simulink model "cart_pole"  (R2024b)
settings: Solver=ode4  StartTime=0.0  StopTime=t_end  FixedStep=0.001  RelTol=1e-3
values from neighbouring files (symbols this model uses):
  alpha = deg2rad(15)    [init_params.m]
  b = 0.1    [init_params.m]    (also in pendulum.m)
  beta = 1.5    [init_params.m]
  C = 0.001    [init_params.m]    (also in pendulum.m = 0.01)
  g = 9.81    [init_params.m]
  J = (1/3)*m*l^2    (= 0.006)    [init_params.m]    (also in pendulum.m)
  K = lqr(A, B, Q, R)    [init_params.m]
  l = 0.3    [init_params.m]    (also in pendulum.m)
  m = 0.2    [init_params.m]    (also in pendulum.m)
  M_t = M_c + m    (= 1.7)    [init_params.m]
  theta0 = pi - 0.05    (= 3.09159265359)    [init_params.m]    (also in pendulum.m = deg2rad(5))
  theta_dot0 = 0    [init_params.m]
  x0 = 0    [init_params.m]    (also in pendulum.m)
  x_dot0 = 0    [init_params.m]
settings Model: Creator=Ali Emir Kaplan  LastModifiedBy=Ali Emir Kaplan

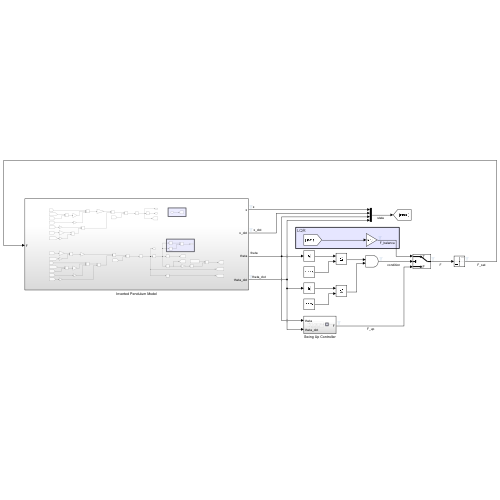
[thumbnail: Simulink's stored preview of the top-level diagram]
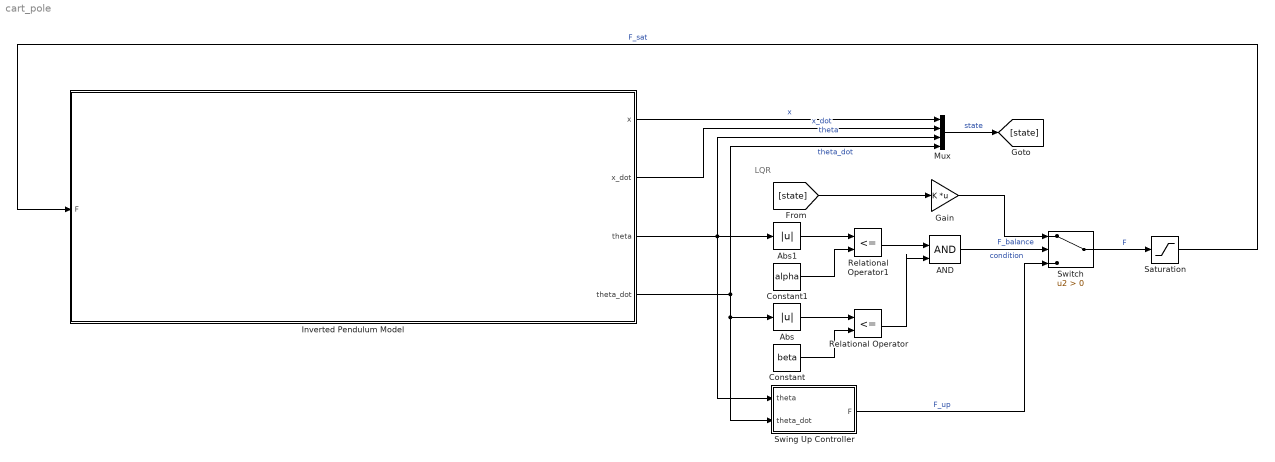
== system cart_pole ==
  note: LQR
  AND : Logic  IconShape=distinctive  AllPortsSameDT=off  OutDataTypeStr=boolean
  Abs : Abs  SaturateOnIntegerOverflow=off
  Abs1 : Abs  SaturateOnIntegerOverflow=off
  Constant : Constant  Value=beta
  Constant1 : Constant  Value=alpha
  Gain : Gain  Gain=K  Multiplication=Matrix(K*u)
  Inverted Pendulum Model : Subsystem
  Mux : Mux
  Relational Operator : RelationalOperator  Operator=<=  OutDataTypeStr=boolean  RndMeth=Simplest  InputSameDT=off
  Relational Operator1 : RelationalOperator  Operator=<=  OutDataTypeStr=boolean  RndMeth=Simplest  InputSameDT=off
  Saturation : Saturate  UpperLimit=+30  LowerLimit=-30
  Swing Up Controller : Subsystem
  Switch : Switch  Criteria=u2 > Threshold  SaturateOnIntegerOverflow=off  InputSameDT=off
  wires:
  Inverted Pendulum Model/1(x) -> Mux/1  "x"
  Inverted Pendulum Model/2(x_dot) -> Mux/2  "x_dot"
  Inverted Pendulum Model/3(theta) -> Mux/3, Abs1/1, Swing Up Controller/1(theta)  "theta"
  Inverted Pendulum Model/4(theta_dot) -> Swing Up Controller/2(theta_dot), Abs/1, Mux/4  "theta_dot"
  Swing Up Controller/1(F) -> Switch/3  "F_up"
  Mux/1 -> [state]  "state"
  [state] -> Gain/1
  Constant/1 -> Relational Operator/2
  Abs/1 -> Relational Operator/1
  Constant1/1 -> Relational Operator1/2
  Abs1/1 -> Relational Operator1/1
  Relational Operator1/1 -> AND/1
  Relational Operator/1 -> AND/2
  Gain/1 -> Switch/1  "F_balance"
  AND/1 -> Switch/2  "condition"
  Switch/1 -> Saturation/1  "F"
  Saturation/1 -> Inverted Pendulum Model/1(F)  "F_sat"

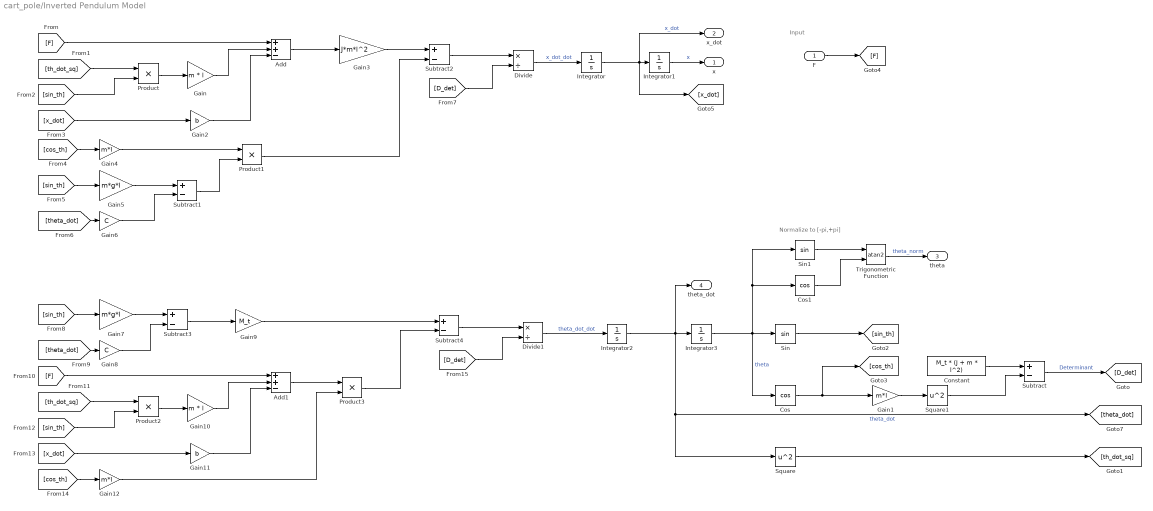
== system cart_pole/Inverted Pendulum Model ==
  note: Input
  note: Normalize to [-pi,+pi]
  F : Inport
  Add : Sum  Inputs=++-
  Add1 : Sum  Inputs=++-
  Constant : Constant  Value=M_t * (J + m * l^2)
  Cos : Trigonometry  Operator=cos
  Cos1 : Trigonometry  Operator=cos
  Divide : Product  Inputs=*/
  Divide1 : Product  Inputs=*/
  Gain : Gain  Gain=m * l
  Gain1 : Gain  Gain=m*l
  Gain10 : Gain  Gain=m * l
  Gain11 : Gain  Gain=b
  Gain12 : Gain  Gain=m*l
  Gain2 : Gain  Gain=b
  Gain3 : Gain  Gain=J*m*l^2
  Gain4 : Gain  Gain=m*l
  Gain5 : Gain  Gain=m*g*l
  Gain6 : Gain  Gain=C
  Gain7 : Gain  Gain=m*g*l
  Gain8 : Gain  Gain=C
  Gain9 : Gain  Gain=M_t
  Integrator : Integrator  InitialCondition=x_dot0
  Integrator1 : Integrator  InitialCondition=x0
  Integrator2 : Integrator  InitialCondition=theta_dot0
  Integrator3 : Integrator  InitialCondition=theta0
  Product{,1..3} (4 alike) : Product
  Sin : Trigonometry
  Sin1 : Trigonometry
  Square : Math  Operator=square
  Square1 : Math  Operator=square
  Subtract{,1..4} (5 alike) : Sum  Inputs=+-
  Trigonometric Function : Trigonometry  Operator=atan2
  x : Outport
  x_dot : Outport  Port=2
  theta : Outport  Port=3
  theta_dot : Outport  Port=4
  wires:
  Integrator1/1 -> x/1  "x"
  Integrator/1 -> x_dot/1, [x_dot], Integrator1/1  "x_dot"
  Divide/1 -> Integrator/1  "x_dot_dot"
  F/1 -> [F]
  [th_dot_sq] -> Product/1
  [sin_th] -> Product/2
  Product/1 -> Gain/1
  Gain/1 -> Add/2
  [F] -> Add/1
  [x_dot] -> Gain2/1
  Gain2/1 -> Add/3
  Add/1 -> Gain3/1
  [cos_th] -> Gain4/1
  [sin_th] -> Gain5/1
  [theta_dot] -> Gain6/1
  Gain5/1 -> Subtract1/1
  Gain6/1 -> Subtract1/2
  Gain4/1 -> Product1/1
  Subtract1/1 -> Product1/2
  Product1/1 -> Subtract2/2
  Gain3/1 -> Subtract2/1
  Subtract2/1 -> Divide/1
  [D_det] -> Divide/2
  [sin_th] -> Gain7/1
  [theta_dot] -> Gain8/1
  Gain7/1 -> Subtract3/1
  Gain8/1 -> Subtract3/2
  Subtract3/1 -> Gain9/1
  Gain11/1 -> Add1/3
  [sin_th] -> Product2/2
  Gain10/1 -> Add1/2
  [F] -> Add1/1
  [th_dot_sq] -> Product2/1
  Product2/1 -> Gain10/1
  [x_dot] -> Gain11/1
  [cos_th] -> Gain12/1
  Add1/1 -> Product3/1
  Gain12/1 -> Product3/2
  Gain9/1 -> Subtract4/1
  Product3/1 -> Subtract4/2
  [D_det] -> Divide1/2
  Subtract4/1 -> Divide1/1
  Divide1/1 -> Integrator2/1  "theta_dot_dot"
  Gain1/1 -> Square1/1
  Integrator2/1 -> theta_dot/1, Square/1, [theta_dot], Integrator3/1  "theta_dot"
  Square/1 -> [th_dot_sq]
  Cos/1 -> [cos_th], Gain1/1
  Integrator3/1 -> Sin1/1, Cos1/1, Cos/1, Sin/1  "theta"
  Constant/1 -> Subtract/1
  Sin/1 -> [sin_th]
  Square1/1 -> Subtract/2
  Subtract/1 -> [D_det]  "Determinant"
  Sin1/1 -> Trigonometric Function/1
  Cos1/1 -> Trigonometric Function/2
  Trigonometric Function/1 -> theta/1  "theta_norm"

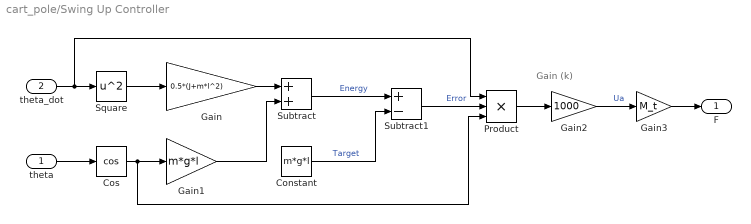
== system cart_pole/Swing Up Controller ==
  note: Gain (k)
  theta : Inport
  theta_dot : Inport  Port=2
  Constant : Constant  Value=m*g*l
  Cos : Trigonometry  Operator=cos
  Gain : Gain  Gain=0.5*(J+m*l^2)
  Gain1 : Gain  Gain=m*g*l
  Gain2 : Gain  Gain=1000
  Gain3 : Gain  Gain=M_t
  Product : Product  Inputs=3
  Square : Math  Operator=square
  Subtract : Sum
  Subtract1 : Sum  Inputs=+-
  F : Outport
  wires:
  Square/1 -> Gain/1
  theta_dot/1 -> Product/1, Square/1
  theta/1 -> Cos/1
  Cos/1 -> Product/3, Gain1/1
  Gain/1 -> Subtract/1
  Gain1/1 -> Subtract/2
  Subtract/1 -> Subtract1/1  "Energy"
  Constant/1 -> Subtract1/2  "Target"
  Subtract1/1 -> Product/2  "Error"
  Product/1 -> Gain2/1
  Gain2/1 -> Gain3/1  "Ua"
  Gain3/1 -> F/1
